simulink model "gm_uz_pmsm_model_9ph_vnl"  (R2021b)
settings: Solver=FixedStepAuto  StartTime=0.0  StopTime=0.8  RelTol=1e-3
PreLoadFcn:
  | uz_pmsm_model_9ph_init_parameter
undefined symbols (not defined in the file or in its folder): a, b, c, friction_coefficient, inertia, k_i_d, k_i_q, k_p_d, k_p_q, Kpd, L_d, L_o1, L_o2, L_q, L_x1, L_x2, L_y1, L_y2, L_zero, polepair, psi_pm, R_1, static_friction_torque, Tnd, ts
libraries: hdlmdlgenlib x191, hdlsllib x90, dspsigops x19, simulink x17, slpidlib x2, spsAlphaBetaZerotodq0Lib x1, pid_lib x1, spsdq0toAlphaBetaZeroLib x1
(part 6 of 7)

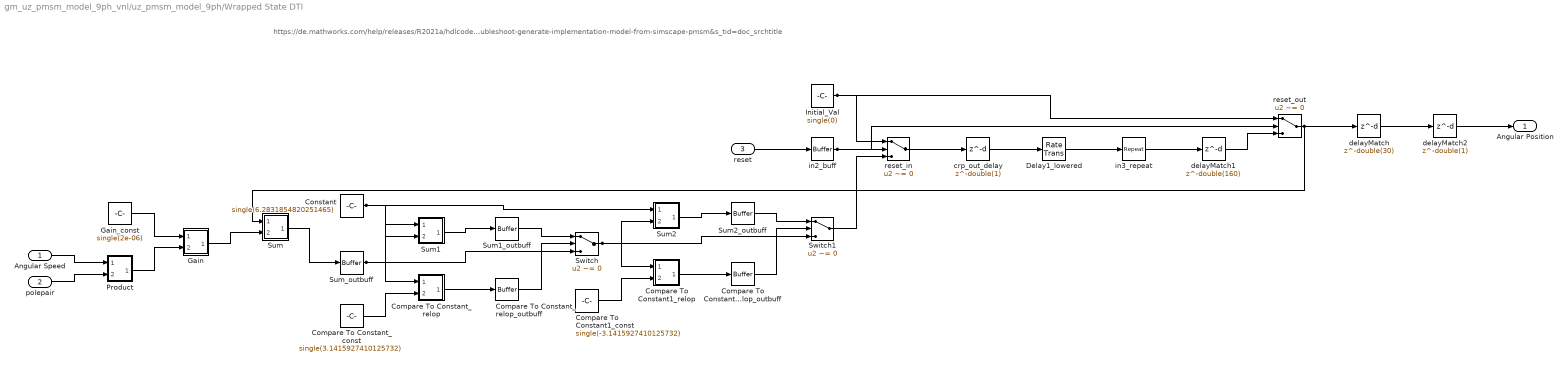
== system gm_uz_pmsm_model_9ph_vnl/uz_pmsm_model_9ph/Wrapped State DTI ==
  note: https://de.mathworks.com/help/releases/R2021a/hdlcoder/ug/troubleshoot-generate-implementation-model-from-simscape-pmsm.html?searchHighlight=troubleshoot-generate-implementation-model-from-simscape-pmsm&s_tid=doc_srchtitle
  Angular Speed : Inport  OutDataTypeStr=single  PortDimensions=1  SampleTime=1e-08
  polepair : Inport  Port=2  OutDataTypeStr=single  PortDimensions=1  SampleTime=1e-08
  reset : Inport  Port=3  OutDataTypeStr=boolean  PortDimensions=1  SampleTime=1e-08
  Compare To Constant1_const : Constant  Value=single(-3.1415927410125732)  OutDataTypeStr=single  SampleTime=1e-08
  Compare To Constant1_relop : Subsystem
      mask Display: disp('NFP\nrelop');
  Compare To Constant1_relop_outbuff : hdlmdlgenlib/Buffer
      settings: SourceProductBaseCode=SL
  Compare To Constant_const : Constant  Value=single(3.1415927410125732)  OutDataTypeStr=single  SampleTime=1e-08
  Compare To Constant_relop : Subsystem
      mask Display: disp('NFP\nrelop');
  Compare To Constant_relop_outbuff : hdlmdlgenlib/Buffer
      settings: SourceProductBaseCode=SL
  Constant : Constant  Value=single(6.2831854820251465)  OutDataTypeStr=single  SampleTime=1e-08
  Delay1_lowered : RateTransition  OutPortSampleTimeOpt=Multiple of input port sample time  OutPortSampleTimeMultiple=200
  Gain : Subsystem
      mask Display: disp('NFP\nmul');
  Gain_const : Constant  Value=single(2e-06)  OutDataTypeStr=single  SampleTime=1e-08
  Initial_Val : Constant  Value=single(0)  OutDataTypeStr=single  SampleTime=1e-08
  Product : Subsystem
      mask Display: disp('NFP\nmul');
  Sum : Subsystem
      mask Display: disp('NFP\nadd');
  Sum1 : Subsystem
      mask Display: disp('NFP\nadd');
  Sum1_outbuff : hdlmdlgenlib/Buffer
      settings: SourceProductBaseCode=SL
  Sum2 : Subsystem
      mask Display: disp('NFP\nadd');
  Sum2_outbuff : hdlmdlgenlib/Buffer
      settings: SourceProductBaseCode=SL
  Sum_outbuff : hdlmdlgenlib/Buffer
      settings: SourceProductBaseCode=SL
  Switch : Switch  Criteria=u2 ~= 0  Threshold=double(0)  OutDataTypeStr=single  SampleTime=1e-08
  Switch1 : Switch  Criteria=u2 ~= 0  Threshold=double(0)  OutDataTypeStr=single  SampleTime=1e-08
  crp_out_delay : Delay  DelayLength=double(1)  InitialCondition=0  SampleTime=1e-08
  delayMatch : Delay  DelayLength=double(30)  InitialCondition=0  SampleTime=1e-08
  delayMatch1 : Delay  DelayLength=double(160)  InitialCondition=0  SampleTime=1e-08
  delayMatch2 : Delay  DelayLength=double(1)  InitialCondition=0  SampleTime=1e-08
  in2_buff : hdlmdlgenlib/Buffer
      settings: SourceProductBaseCode=SL
  in3_repeat : dspsigops/Repeat  N=double(200)  RateOptions=Allow multirate processing  ic=0  mode=Unused parameter value
  reset_in : Switch  Criteria=u2 ~= 0  Threshold=double(0)  OutDataTypeStr=single  SampleTime=1e-08
  reset_out : Switch  Criteria=u2 ~= 0  Threshold=double(0)  OutDataTypeStr=single  SampleTime=1e-08
  Angular Position : Outport  SampleTime=1e-08
  wires:
  delayMatch/1 -> delayMatch2/1
  reset_out/1 -> Sum/1(In1), delayMatch/1
  Switch/1 -> Switch1/3, Compare To Constant1_relop/1(In1), Sum2/2(In2)
  Compare To Constant1_relop_outbuff/1 -> Switch1/2
  Sum_outbuff/1 -> Switch/3, Sum1/1(In1), Compare To Constant_relop/1(In1)
  Compare To Constant_relop_outbuff/1 -> Switch/2
  delayMatch1/1 -> reset_out/3
  in2_buff/1 -> reset_in/2, reset_out/2
  Gain/1(Out1) -> Sum/2(In2)
  Compare To Constant_relop/1(Out1) -> Compare To Constant_relop_outbuff/1
  Sum2/1(Out1) -> Sum2_outbuff/1
  Compare To Constant1_relop/1(Out1) -> Compare To Constant1_relop_outbuff/1
  Sum/1(Out1) -> Sum_outbuff/1
  Product/1(Out1) -> Gain/2(In2)
  Sum1/1(Out1) -> Sum1_outbuff/1
  Gain_const/1 -> Gain/1(In1)
  Compare To Constant_const/1 -> Compare To Constant_relop/2(In2)
  Compare To Constant1_const/1 -> Compare To Constant1_relop/2(In2)
  reset_in/1 -> crp_out_delay/1
  Sum2_outbuff/1 -> Switch1/1
  Switch1/1 -> reset_in/3
  Initial_Val/1 -> reset_in/1, reset_out/1
  Sum1_outbuff/1 -> Switch/1
  Constant/1 -> Sum1/2(In2), Sum2/1(In1)
  delayMatch2/1 -> Angular Position/1
  in3_repeat/1 -> delayMatch1/1
  crp_out_delay/1 -> Delay1_lowered/1
  Delay1_lowered/1 -> in3_repeat/1
  reset/1 -> in2_buff/1
  polepair/1 -> Product/2(In2)
  Angular Speed/1 -> Product/1(In1)

== system gm_uz_pmsm_model_9ph_vnl/uz_pmsm_model_9ph_vnl/Line-Line to Phase voltage ==
  In1 : Inport
  Complex to Real-Imag : ComplexToRealImag
  Constant : Constant  Value=0  OutDataTypeStr=single  SampleTime=ts
  Constant1 : Constant  Value=1/sqrt(3)*exp(1i*-30/180*pi)  OutDataTypeStr=single  SampleTime=ts
  Demux3 : Demux  Outputs=3
  Mux4 : Mux  Inputs=3
  Product : Product  OutDataTypeStr=single
  Real-Imag to Complex : RealImagToComplex
  Terminator : Terminator
  abc   to   alpha_beta_0 : Subsystem
  alpha_beta_0   to   abc : Subsystem
  Out1 : Outport
  wires:
  Constant1/1 -> Product/2
  alpha_beta_0   to   abc/1("a, b, c") -> Out1/1
  abc   to   alpha_beta_0/1("alpha, beta, 0 ") -> Demux3/1
  Demux3/3 -> Terminator/1
  In1/1 -> abc   to   alpha_beta_0/1("a, b, c")
  Constant/1 -> Mux4/3
  Complex to Real-Imag/2 -> Mux4/2
  Demux3/1 -> Real-Imag to Complex/1
  Real-Imag to Complex/1 -> Product/1
  Product/1 -> Complex to Real-Imag/1
  Mux4/1 -> alpha_beta_0   to   abc/1("alpha, beta, 0  ")
  Complex to Real-Imag/1 -> Mux4/1
  Demux3/2 -> Real-Imag to Complex/2

== system gm_uz_pmsm_model_9ph_vnl/uz_pmsm_model_9ph_vnl/Line-Line to Phase voltage1 ==
  In1 : Inport
  Complex to Real-Imag : ComplexToRealImag
  Constant : Constant  Value=0  OutDataTypeStr=single  SampleTime=ts
  Constant1 : Constant  Value=1/sqrt(3)*exp(1i*-30/180*pi)  OutDataTypeStr=single  SampleTime=ts
  Demux3 : Demux  Outputs=3
  Mux4 : Mux  Inputs=3
  Product : Product  OutDataTypeStr=single
  Real-Imag to Complex : RealImagToComplex
  Terminator : Terminator
  abc   to   alpha_beta_0 : Subsystem
  alpha_beta_0   to   abc : Subsystem
  Out1 : Outport
  wires:
  Demux3/2 -> Real-Imag to Complex/2
  Complex to Real-Imag/1 -> Mux4/1
  Mux4/1 -> alpha_beta_0   to   abc/1("alpha, beta, 0  ")
  Product/1 -> Complex to Real-Imag/1
  Real-Imag to Complex/1 -> Product/1
  Demux3/1 -> Real-Imag to Complex/1
  Complex to Real-Imag/2 -> Mux4/2
  Constant/1 -> Mux4/3
  In1/1 -> abc   to   alpha_beta_0/1("a, b, c")
  Demux3/3 -> Terminator/1
  abc   to   alpha_beta_0/1("alpha, beta, 0 ") -> Demux3/1
  alpha_beta_0   to   abc/1("a, b, c") -> Out1/1
  Constant1/1 -> Product/2

== system gm_uz_pmsm_model_9ph_vnl/uz_pmsm_model_9ph_vnl/Line-Line to Phase voltage2 ==
  In1 : Inport
  Complex to Real-Imag : ComplexToRealImag
  Constant : Constant  Value=0  OutDataTypeStr=single  SampleTime=ts
  Constant1 : Constant  Value=1/sqrt(3)*exp(1i*-30/180*pi)  OutDataTypeStr=single  SampleTime=ts
  Demux3 : Demux  Outputs=3
  Mux4 : Mux  Inputs=3
  Product : Product  OutDataTypeStr=single
  Real-Imag to Complex : RealImagToComplex
  Terminator : Terminator
  abc   to   alpha_beta_0 : Subsystem
  alpha_beta_0   to   abc : Subsystem
  Out1 : Outport
  wires:
  Constant1/1 -> Product/2
  alpha_beta_0   to   abc/1("a, b, c") -> Out1/1
  abc   to   alpha_beta_0/1("alpha, beta, 0 ") -> Demux3/1
  Demux3/3 -> Terminator/1
  In1/1 -> abc   to   alpha_beta_0/1("a, b, c")
  Constant/1 -> Mux4/3
  Complex to Real-Imag/2 -> Mux4/2
  Demux3/1 -> Real-Imag to Complex/1
  Real-Imag to Complex/1 -> Product/1
  Product/1 -> Complex to Real-Imag/1
  Mux4/1 -> alpha_beta_0   to   abc/1("alpha, beta, 0  ")
  Complex to Real-Imag/1 -> Mux4/1
  Demux3/2 -> Real-Imag to Complex/2

== system gm_uz_pmsm_model_9ph_vnl/uz_pmsm_model_9ph_vnl/Transformation ==
  in : Inport
  Add : Sum
  Add1 : Sum  Inputs=-+
  Constant1 : Constant  Value=c  OutDataTypeStr=fixdt(1,18)  SampleTime=ts
  Data Type Conversion1 : DataTypeConversion  OutDataTypeStr=single  RndMeth=Nearest
  Data Type Conversion38 : DataTypeConversion  OutDataTypeStr=single  RndMeth=Nearest
  Data Type Conversion39 : DataTypeConversion  OutDataTypeStr=single  RndMeth=Nearest
  Demux1 : Demux  Outputs=9
  Divide{,1..3} (4 alike) : Product  Inputs=**
  MatrixMultiply : Product  Multiplication=Matrix(*)
  Mux : Mux  Inputs=9
  out : Outport
  wires:
  in/1 -> MatrixMultiply/2
  Data Type Conversion39/1 -> Demux1/1
  Constant1/1 -> MatrixMultiply/1
  MatrixMultiply/1 -> Data Type Conversion39/1
  Divide2/1 -> Add1/1
  Divide3/1 -> Add1/2
  [cos_theta_el] -> Divide3/1
  [sin_theta_el] -> Divide2/1
  [cos_theta_el] -> Divide/1  "cos_theta_hdl"
  [sin_theta_el] -> Divide1/1  "sin_theta_hdl"
  Divide1/1 -> Add/2
  Divide/1 -> Add/1
  Data Type Conversion1/1 -> Divide3/2, Divide1/2  "u_beta"
  Data Type Conversion38/1 -> Divide2/2, Divide/2  "u_alpha"
  Add/1 -> Mux/1
  Add1/1 -> Mux/2
  Demux1/2 -> Data Type Conversion1/1
  Demux1/1 -> Data Type Conversion38/1
  Mux/1 -> out/1  "trafo_out"
  Demux1/9 -> Mux/9
  Demux1/8 -> Mux/8
  Demux1/7 -> Mux/7
  Demux1/6 -> Mux/6
  Demux1/5 -> Mux/5
  Demux1/4 -> Mux/4
  Demux1/3 -> Mux/3

== system gm_uz_pmsm_model_9ph_vnl/uz_pmsm_model_9ph_vnl/Transformation1 ==
  in : Inport
  Add : Sum  Inputs=+-
  Add1 : Sum
  Constant1 : Constant  Value=inv(c)  OutDataTypeStr=fixdt(1,18)  SampleTime=ts
  Data Type Conversion28 : DataTypeConversion  OutDataTypeStr=fixdt(1,25,12)  RndMeth=Nearest
  Demux1 : Demux  Outputs=9
  Divide{,1..3} (4 alike) : Product  Inputs=**
  MatrixMultiply : Product  Multiplication=Matrix(*)
  Mux : Mux  Inputs=9
  out : Outport
  wires:
  MatrixMultiply/1 -> out/1
  Constant1/1 -> MatrixMultiply/1
  Data Type Conversion28/1 -> MatrixMultiply/2
  Add1/1 -> Mux/2
  [cos_theta_el] -> Divide3/1
  Divide2/1 -> Add1/1
  [sin_theta_el] -> Divide2/1
  Divide3/1 -> Add1/2
  Demux1/1 -> Divide/2, Divide2/2  "i_d"
  Divide1/1 -> Add/2
  [cos_theta_el] -> Divide/1
  Divide/1 -> Add/1
  Add/1 -> Mux/1
  Demux1/2 -> Divide1/2, Divide3/2  "i_q"
  [sin_theta_el] -> Divide1/1
  Demux1/7 -> Mux/7
  Demux1/9 -> Mux/9
  Demux1/5 -> Mux/5
  Demux1/3 -> Mux/3
  Demux1/4 -> Mux/4
  Demux1/6 -> Mux/6
  Demux1/8 -> Mux/8
  Mux/1 -> Data Type Conversion28/1
  in/1 -> Demux1/1

== system gm_uz_pmsm_model_9ph_vnl/uz_pmsm_model_9ph_vnl/Wrapped State DTI ==
  note: https://de.mathworks.com/help/releases/R2021a/hdlcoder/ug/troubleshoot-generate-implementation-model-from-simscape-pmsm.html?searchHighlight=troubleshoot-generate-implementation-model-from-simscape-pmsm&s_tid=doc_srchtitle
  Angular Speed : Inport
  polepair : Inport  Port=2
  reset : Inport  Port=3
  Compare To Constant : simulink/Logic and Bit Operations/Compare To Constant  relop=>=  const=single(pi)  OutDataTypeStr=boolean
  Compare To Constant1 : simulink/Logic and Bit Operations/Compare To Constant  relop=<  const=single(-pi)  OutDataTypeStr=boolean
  Constant : Constant  Value=single(2*pi)  SampleTime=-1
  Delay1 : Delay  DelayLength=1  ExternalReset=Level
      settings: InputPortMap=u0,r5
  Gain : Gain  Gain=ts
  Product : Product
  Sum : Sum  Inputs=|++
  Sum1 : Sum  Inputs=|-+
  Sum2 : Sum  Inputs=|++
  Switch : Switch  Criteria=u2 > Threshold
  Switch1 : Switch  Criteria=u2 > Threshold
  Angular Position : Outport
  wires:
  polepair/1 -> Product/2
  Angular Speed/1 -> Product/1
  Product/1 -> Gain/1
  reset/1 -> Delay1/2
  Gain/1 -> Sum/2
  Sum1/1 -> Switch/1
  Sum/1 -> Switch/3, Sum1/2, Compare To Constant/1
  Compare To Constant/1 -> Switch/2
  Switch/1 -> Switch1/3, Compare To Constant1/1, Sum2/2
  Switch1/1 -> Delay1/1  "Angular Position"
  Sum2/1 -> Switch1/1
  Constant/1 -> Sum1/1, Sum2/1
  Delay1/1 -> Angular Position/1, Sum/1
  Compare To Constant1/1 -> Switch1/2

== system gm_uz_pmsm_model_9ph_vnl/uz_pmsm_model_9ph_vnl/mechanical_system ==
  note: This delay breaks the algebraic loop between mechanical and electrical system.
      | Introduces a delay of 500ns.
  note: load torque negative!!!
  reset : Inport
  M_Mi : Inport  Port=2
  reciprocal_J : Inport  Port=3
  load_torque : Inport  Port=4
  Data Type Conversion1 : DataTypeConversion  OutDataTypeStr=double  RndMeth=Nearest
  Data Type Conversion8 : DataTypeConversion  OutDataTypeStr=single  RndMeth=Nearest
  Delay : Delay  DelayLength=1
  Product11 : Product
  Sum1 : Sum  Inputs=|++
  integrator : Subsystem
  omega_mech : Outport
  wires:
  reset/1 -> integrator/2(reset)
  Data Type Conversion1/1 -> integrator/1(in)
  Data Type Conversion8/1 -> omega_mech/1
  Delay/1 -> Sum1/1
  M_Mi/1 -> Delay/1
  load_torque/1 -> Sum1/2
  Sum1/1 -> Product11/2
  reciprocal_J/1 -> Product11/1
  integrator/1(outt) -> Data Type Conversion8/1
  Product11/1 -> Data Type Conversion1/1

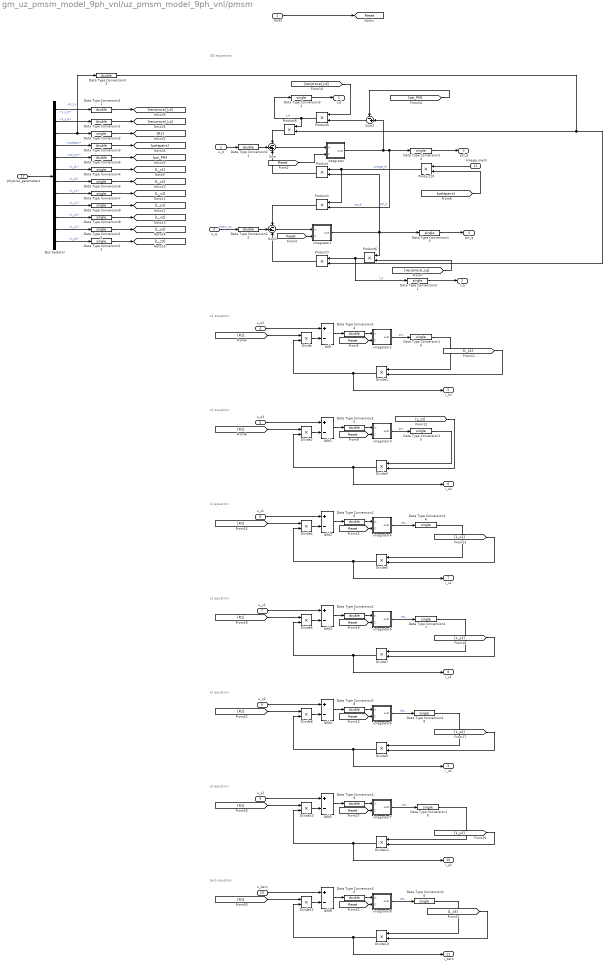
== system gm_uz_pmsm_model_9ph_vnl/uz_pmsm_model_9ph_vnl/pmsm ==
  note: zero equation
  note: y2 equation
  note: x2 equation
  note: y1 equation
  note: x1 equation
  note: o2 equation
  note: DQ equations
  note: o1 equation
  reset : Inport
  u_d : Inport  Port=2
  u_q : Inport  Port=3
  u_o1 : Inport  Port=4
  u_o2 : Inport  Port=5
  u_x1 : Inport  Port=6
  u_y1 : Inport  Port=7
  u_x2 : Inport  Port=8
  u_y2 : Inport  Port=9
  u_zero : Inport  Port=10
  omega_mech : Inport  Port=11
  physical_parameters : Inport  Port=12
  Add{,1..6} (7 alike) : Sum  Inputs=+-
  Bus Selector : BusSelector  OutputSignals=1_L_d,1_L_q,R_1,polepair,psi_pm,L_z1,L_z2,L_x1,L_y1,L_x2,L_y2,L_z3
  Data Type Conversion{1,3,5,11,21..22,24..30,33} (14 alike) : DataTypeConversion  OutDataTypeStr=double  RndMeth=Nearest
  Data Type Conversion{2,4,6..10,12..20,23,31..32} (19 alike) : DataTypeConversion  OutDataTypeStr=single  RndMeth=Nearest
  Divide{,1..13} (14 alike) : Product  Inputs=**
  Product{,1,5..8,10} (7 alike) : Product
  Sum : Sum  Inputs=-++
  Sum1 : Sum  Inputs=-+-
  Sum2 : Sum  Inputs=-+|
  integrator : Subsystem
  integrator1 : Subsystem
  integrator2 : Subsystem
  integrator3 : Subsystem
  integrator4 : Subsystem
  integrator5 : Subsystem
  integrator6 : Subsystem
  integrator7 : Subsystem
  integrator8 : Subsystem
  I_d : Outport
  I_q : Outport  Port=2
  psi_d : Outport  Port=3
  psi_q : Outport  Port=4
  i_o1 : Outport  Port=5
  i_o2 : Outport  Port=6
  i_x1 : Outport  Port=7
  i_y1 : Outport  Port=8
  i_x2 : Outport  Port=9
  i_y2 : Outport  Port=10
  i_zero : Outport  Port=11
  tag scope: Reset=global
  wires:
  Data Type Conversion32/1 -> I_d/1
  Data Type Conversion23/1 -> psi_d/1
  Data Type Conversion21/1 -> Sum/2
  Data Type Conversion31/1 -> I_q/1
  Data Type Conversion13/1 -> psi_q/1
  Data Type Conversion22/1 -> Sum1/2
  Data Type Conversion30/1 -> integrator8/1(in)
  Data Type Conversion29/1 -> integrator7/1(in)
  Data Type Conversion28/1 -> integrator6/1(in)
  Data Type Conversion27/1 -> integrator5/1(in)
  Data Type Conversion26/1 -> integrator4/1(in)
  Data Type Conversion25/1 -> integrator3/1(in)
  Data Type Conversion24/1 -> integrator2/1(in)
  Sum1/1 -> integrator1/1(in)
  Sum/1 -> integrator/1(in)
  Data Type Conversion20/1 -> Divide13/1
  Data Type Conversion19/1 -> Divide11/1
  Data Type Conversion18/1 -> Divide9/1
  Data Type Conversion17/1 -> Divide7/1
  Data Type Conversion16/1 -> Divide5/1
  Data Type Conversion15/1 -> Divide3/1
  Data Type Conversion14/1 -> Divide1/1
  [L_z3] -> Divide13/2
  [L_y2] -> Divide11/2
  [L_x2] -> Divide9/2
  [L_y1] -> Divide7/2
  [L_x1] -> Divide5/2
  [polepairs] -> Product10/2
  Data Type Conversion2/1 -> [R1]
  Bus Selector/9 -> Data Type Conversion9/1  "<L_y1>"
  Data Type Conversion11/1 -> [reciprocal_Ld]
  Data Type Conversion3/1 -> [polepairs]
  physical_parameters/1 -> Bus Selector/1
  Data Type Conversion4/1 -> [L_z1]
  Bus Selector/10 -> Data Type Conversion8/1  "<L_x2>"
  Bus Selector/3 -> Data Type Conversion2/1, Data Type Conversion33/1  "<R_1>"
  Bus Selector/12 -> Data Type Conversion12/1  "<L_z3>"
  Bus Selector/11 -> Data Type Conversion10/1  "<L_y2>"
  Data Type Conversion6/1 -> [L_z2]
  Data Type Conversion7/1 -> [L_x1]
  Bus Selector/7 -> Data Type Conversion6/1  "<L_z2>"
  Bus Selector/6 -> Data Type Conversion4/1  "<L_z1>"
  Data Type Conversion10/1 -> [L_y2]
  Data Type Conversion8/1 -> [L_x2]
  Bus Selector/5 -> Data Type Conversion5/1  "<psi_pm>"
  Bus Selector/2 -> Data Type Conversion1/1  "<1_L_q>"
  Bus Selector/8 -> Data Type Conversion7/1  "<L_x1>"
  Bus Selector/4 -> Data Type Conversion3/1  "<polepair>"
  Data Type Conversion5/1 -> [psi_PM]
  Data Type Conversion1/1 -> [reciprocal_Lq]
  Data Type Conversion9/1 -> [L_y1]
  Data Type Conversion12/1 -> [L_z3]
  Bus Selector/1 -> Data Type Conversion11/1  "<1_L_d>"
  integrator8/1(outt) -> Data Type Conversion20/1  "psi_"
  [R1] -> Divide12/1
  Add6/1 -> Data Type Conversion30/1
  Divide12/1 -> Add6/2
  Divide13/1 -> Divide12/2, i_zero/1
  u_zero/1 -> Add6/1
  [Reset] -> integrator8/2(reset)
  [Reset] -> integrator7/2(reset)
  u_y2/1 -> Add5/1
  Divide11/1 -> Divide10/2, i_y2/1
  Divide10/1 -> Add5/2
  Add5/1 -> Data Type Conversion29/1
  [R1] -> Divide10/1
  integrator7/1(outt) -> Data Type Conversion19/1  "psi_"
  integrator6/1(outt) -> Data Type Conversion18/1  "psi_"
  [R1] -> Divide8/1
  Add4/1 -> Data Type Conversion28/1
  Divide8/1 -> Add4/2
  Divide9/1 -> Divide8/2, i_x2/1
  u_x2/1 -> Add4/1
  [Reset] -> integrator6/2(reset)
  [Reset] -> integrator5/2(reset)
  u_y1/1 -> Add3/1
  Divide7/1 -> Divide6/2, i_y1/1
  Divide6/1 -> Add3/2
  Add3/1 -> Data Type Conversion27/1
  [R1] -> Divide6/1
  integrator5/1(outt) -> Data Type Conversion17/1  "psi_"
  integrator4/1(outt) -> Data Type Conversion16/1  "psi_"
  [R1] -> Divide4/1
  Add2/1 -> Data Type Conversion26/1
  Divide4/1 -> Add2/2
  Divide5/1 -> Divide4/2, i_x1/1
  u_x1/1 -> Add2/1
  [Reset] -> integrator4/2(reset)
  [Reset] -> integrator3/2(reset)
  [L_z2] -> Divide3/2
  u_o2/1 -> Add1/1
  Divide3/1 -> Divide2/2, i_o2/1
  Divide2/1 -> Add1/2
  Add1/1 -> Data Type Conversion25/1
  [R1] -> Divide2/1
  integrator3/1(outt) -> Data Type Conversion15/1  "psi_"
  integrator2/1(outt) -> Data Type Conversion14/1  "psi_"
  [R1] -> Divide/1
  Add/1 -> Data Type Conversion24/1
  Divide/1 -> Add/2
  Divide1/1 -> Divide/2, i_o1/1
  u_o1/1 -> Add/1
  [L_z1] -> Divide1/2
  [Reset] -> integrator2/2(reset)
  [Reset] -> integrator1/2(reset)
  [Reset] -> integrator/2(reset)
  reset/1 -> [Reset]
  Data Type Conversion33/1 -> Product7/2, Product8/2
  Product7/1 -> Sum1/3
  [reciprocal_Lq] -> Product6/2
  Product8/1 -> Sum/1
  Sum2/1 -> Product5/2
  integrator/1(outt) -> Data Type Conversion23/1, Product1/2, Sum2/2  "psi_d"
  Product10/1 -> Product/1, Product1/1  "omega_el"
  Product6/1 -> Product7/1, Data Type Conversion31/1  "I_q"
  [psi_PM] -> Sum2/1
  Product1/1 -> Sum1/1
  u_d/1 -> Data Type Conversion21/1
  integrator1/1(outt) -> Product6/1, Product/2, Data Type Conversion13/1  "psi_q"
  [reciprocal_Ld] -> Product5/1
  Product5/1 -> Product8/1, Data Type Conversion32/1  "I_d"
  Product/1 -> Sum/3
  u_q/1 -> Data Type Conversion22/1  "intern_uq"
  omega_mech/1 -> Product10/1

== system gm_uz_pmsm_model_9ph_vnl/uz_pmsm_model_9ph_vnl/torque_calculation ==
  I_d : Inport
  I_q : Inport  Port=2
  psi_d : Inport  Port=3
  psi_q : Inport  Port=4
  polepairs : Inport  Port=5
  Factor : Gain  Gain=9/2
  Product2 : Product
  Product3 : Product
  Product9 : Product
  Sum3 : Sum  Inputs=-|+
  M_Mi : Outport
  wires:
  Factor/1 -> Product9/1  "M_Mi"
  polepairs/1 -> Product9/2
  Product9/1 -> M_Mi/1  "M_Mi"
  I_q/1 -> Product3/2
  I_d/1 -> Product2/1
  psi_d/1 -> Product3/1
  psi_q/1 -> Product2/2
  Product2/1 -> Sum3/1
  Product3/1 -> Sum3/2
  Sum3/1 -> Factor/1

== system gm_uz_pmsm_model_9ph_vnl/Compare/Assert_i_abc_ps/RelErrCheck ==
  In1 : Inport
  In2 : Inport  Port=2
  "RelativeErrorCheck " : MATLAB Function  TreatAsAtomicUnit=on
  Out1 : Outport  VectorParamsAs1DForOutWhenUnconnected=off
  wires:
  "RelativeErrorCheck "/1(y) -> Out1/1
  In1/1 -> "RelativeErrorCheck "/1(P)
  In2/1 -> "RelativeErrorCheck "/2(R)

== system gm_uz_pmsm_model_9ph_vnl/Compare/Assert_outputs/RelErrCheck ==
  In1 : Inport
  In2 : Inport  Port=2
  "RelativeErrorCheck " : MATLAB Function  TreatAsAtomicUnit=on
  Out1 : Outport  VectorParamsAs1DForOutWhenUnconnected=off
  wires:
  "RelativeErrorCheck "/1(y) -> Out1/1
  In1/1 -> "RelativeErrorCheck "/1(P)
  In2/1 -> "RelativeErrorCheck "/2(R)

== system gm_uz_pmsm_model_9ph_vnl/uz_pmsm_model_9ph/Line-Line to Phase voltage/Product ==
  In1 : Inport
  In2 : Inport  Port=2
  Product : Product  Inputs=**  OutDataTypeStr=single  SampleTime=1e-08
  Product_pd1 : Delay  DelayLength=6
  Out1 : Outport
  wires:
  Product_pd1/1 -> Out1/1
  Product/1 -> Product_pd1/1
  In2/1 -> Product/2
  In1/1 -> Product/1

== system gm_uz_pmsm_model_9ph_vnl/uz_pmsm_model_9ph/Line-Line to Phase voltage/Product1 ==
  In1 : Inport
  In2 : Inport  Port=2
  Product1 : Product  Inputs=**  OutDataTypeStr=single  SampleTime=1e-08
  Product1_pd1 : Delay  DelayLength=6
  Out1 : Outport
  wires:
  Product1_pd1/1 -> Out1/1
  Product1/1 -> Product1_pd1/1
  In2/1 -> Product1/2
  In1/1 -> Product1/1

== system gm_uz_pmsm_model_9ph_vnl/uz_pmsm_model_9ph/Line-Line to Phase voltage/Product2 ==
  In1 : Inport
  In2 : Inport  Port=2
  Product2 : Product  Inputs=**  OutDataTypeStr=single  SampleTime=1e-08
  Product2_pd1 : Delay  DelayLength=6
  Out1 : Outport
  wires:
  Product2_pd1/1 -> Out1/1
  Product2/1 -> Product2_pd1/1
  In2/1 -> Product2/2
  In1/1 -> Product2/1

== system gm_uz_pmsm_model_9ph_vnl/uz_pmsm_model_9ph/Line-Line to Phase voltage/Product3 ==
  In1 : Inport
  In2 : Inport  Port=2
  Product3 : Product  Inputs=**  OutDataTypeStr=single  SampleTime=1e-08
  Product3_pd1 : Delay  DelayLength=6
  Out1 : Outport
  wires:
  Product3_pd1/1 -> Out1/1
  Product3/1 -> Product3_pd1/1
  In2/1 -> Product3/2
  In1/1 -> Product3/1

== system gm_uz_pmsm_model_9ph_vnl/uz_pmsm_model_9ph/Line-Line to Phase voltage/Product_AC_minus_BD ==
  In1 : Inport
  In2 : Inport  Port=2
  Product_AC_minus_BD : Sum  Inputs=+-  OutDataTypeStr=single  SampleTime=1e-08
  Product_AC_minus_BD_pd1 : Delay  DelayLength=6
  Out1 : Outport
  wires:
  Product_AC_minus_BD_pd1/1 -> Out1/1
  Product_AC_minus_BD/1 -> Product_AC_minus_BD_pd1/1
  In2/1 -> Product_AC_minus_BD/2
  In1/1 -> Product_AC_minus_BD/1

== system gm_uz_pmsm_model_9ph_vnl/uz_pmsm_model_9ph/Line-Line to Phase voltage/Product_AD_plus_BC ==
  In1 : Inport
  In2 : Inport  Port=2
  Product_AD_plus_BC : Sum  OutDataTypeStr=single  SampleTime=1e-08
  Product_AD_plus_BC_pd1 : Delay  DelayLength=6
  Out1 : Outport
  wires:
  Product_AD_plus_BC_pd1/1 -> Out1/1
  Product_AD_plus_BC/1 -> Product_AD_plus_BC_pd1/1
  In2/1 -> Product_AD_plus_BC/2
  In1/1 -> Product_AD_plus_BC/1

== system gm_uz_pmsm_model_9ph_vnl/uz_pmsm_model_9ph/Line-Line to Phase voltage/abc   to   alpha_beta_0 ==
  "a, b, c" : Inport  OutDataTypeStr=single  PortDimensions=[3]  SampleTime=1e-08
  Gain2 : Subsystem
      mask Display: disp('NFP\nmul');
  Gain2_const : Constant  Value=single(0.6666666865348816)  OutDataTypeStr=single  SampleTime=1e-08
  Gain4_const : Constant  Value=single([1 0 0.5 -0.5 0.8660253882408142 0.5 -0.5 -0.8660253882408142 0.5]).'  OutDataTypeStr=single  SampleTime=1e-08
  MMul_add_01 : Subsystem
      mask Display: disp('NFP\nadd');
  MMul_add_12 : Subsystem
      mask Display: disp('NFP\nadd');
  MMul_dot_product : Subsystem
      mask Display: disp('NFP\nmul');
  Reshape : Reshape  OutputDimensionality=Column vector (2-D)
  Row2Col_in0 : Reshape  OutputDimensionality=Column vector (2-D)
  Row2Col_in1 : Reshape  OutputDimensionality=Column vector (2-D)
  delayMatch : Delay  DelayLength=double(6)  InitialCondition=0  SampleTime=1e-08
  delayMatch1 : Delay  DelayLength=double(18)  InitialCondition=0  SampleTime=1e-08
  reshape_dotProduct : Reshape  OutputDimensionality=Customize  OutputDimensions=[3,3]
  reshape_mmulResult : Reshape  OutputDimensionality=Customize  OutputDimensions=[3,1]
  select_0 : Selector  NumberOfDimensions=2  SampleTime=1e-08  IndexOptions=Index vector (dialog),Select all  Indices=double(1),[]  OutputSizes=1
  select_1 : Selector  NumberOfDimensions=2  SampleTime=1e-08  IndexOptions=Index vector (dialog),Select all  Indices=double(2),[]  OutputSizes=1
  select_2 : Selector  NumberOfDimensions=2  SampleTime=1e-08  IndexOptions=Index vector (dialog),Select all  Indices=double(3),[]  OutputSizes=1
  select_indices0 : Selector  SampleTime=1e-08  IndexOptions=Index vector (dialog)  Indices=double([1 4 7 2 5 8 3 6 9])  OutputSizes=1
  select_indices1 : Selector  SampleTime=1e-08  IndexOptions=Index vector (dialog)  Indices=double([1 2 3 1 2 3 1 2 3])  OutputSizes=1
  t : Reshape  OutputDimensionality=Customize  OutputDimensions=[3,3]
  t1 : Mux  Inputs=3
  vectorized_in0 : Reshape  OutputDimensionality=Row vector (2-D)
  "alpha, beta, 0 " : Outport  SampleTime=1e-08
  wires:
  "a, b, c"/1 -> Reshape/1
  t1/1 -> delayMatch1/1
  select_2/1 -> delayMatch/1
  Gain2/1(Out1) -> "alpha, beta, 0 "/1
  delayMatch1/1 -> Gain2/2(In2)
  MMul_add_12/1(Out1) -> reshape_mmulResult/1
  MMul_add_01/1(Out1) -> MMul_add_12/1(In1)
  MMul_dot_product/1(Out1) -> reshape_dotProduct/1
  Gain2_const/1 -> t1/1, t1/2, t1/3
  Gain4_const/1 -> t/1
  delayMatch/1 -> MMul_add_12/2(In2)
  select_1/1 -> MMul_add_01/2(In2)
  select_0/1 -> MMul_add_01/1(In1)
  reshape_dotProduct/1 -> select_0/1, select_1/1, select_2/1
  Row2Col_in1/1 -> MMul_dot_product/2(In2)
  Row2Col_in0/1 -> MMul_dot_product/1(In1)
  select_indices1/1 -> Row2Col_in1/1
  select_indices0/1 -> Row2Col_in0/1
  vectorized_in0/1 -> select_indices0/1
  t/1 -> vectorized_in0/1
  Reshape/1 -> select_indices1/1
  reshape_mmulResult/1 -> Gain2/1(In1)

== system gm_uz_pmsm_model_9ph_vnl/uz_pmsm_model_9ph/Line-Line to Phase voltage/alpha_beta_0   to   abc ==
  "alpha, beta, 0  " : Inport  OutDataTypeStr=single  PortDimensions=[3]  SampleTime=1e-08
  Gain4_const : Constant  Value=single([1 -0.5 -0.5 0 0.8660253882408142 -0.8660253882408142 1 1 1]).'  OutDataTypeStr=single  SampleTime=1e-08
  MMul_add_01 : Subsystem
      mask Display: disp('NFP\nadd');
  MMul_add_12 : Subsystem
      mask Display: disp('NFP\nadd');
  MMul_dot_product : Subsystem
      mask Display: disp('NFP\nmul');
  Reshape : Reshape  OutputDimensionality=Column vector (2-D)
  Row2Col_in0 : Reshape  OutputDimensionality=Column vector (2-D)
  Row2Col_in1 : Reshape  OutputDimensionality=Column vector (2-D)
  delayMatch : Delay  DelayLength=double(6)  InitialCondition=0  SampleTime=1e-08
  reshape_dotProduct : Reshape  OutputDimensionality=Customize  OutputDimensions=[3,3]
  reshape_mmulResult : Reshape  OutputDimensionality=Customize  OutputDimensions=[3,1]
  select_0 : Selector  NumberOfDimensions=2  SampleTime=1e-08  IndexOptions=Index vector (dialog),Select all  Indices=double(1),[]  OutputSizes=1
  select_1 : Selector  NumberOfDimensions=2  SampleTime=1e-08  IndexOptions=Index vector (dialog),Select all  Indices=double(2),[]  OutputSizes=1
  select_2 : Selector  NumberOfDimensions=2  SampleTime=1e-08  IndexOptions=Index vector (dialog),Select all  Indices=double(3),[]  OutputSizes=1
  select_indices0 : Selector  SampleTime=1e-08  IndexOptions=Index vector (dialog)  Indices=double([1 4 7 2 5 8 3 6 9])  OutputSizes=1
  select_indices1 : Selector  SampleTime=1e-08  IndexOptions=Index vector (dialog)  Indices=double([1 2 3 1 2 3 1 2 3])  OutputSizes=1
  t : Reshape  OutputDimensionality=Customize  OutputDimensions=[3,3]
  vectorized_in0 : Reshape  OutputDimensionality=Row vector (2-D)
  "a, b, c" : Outport  SampleTime=1e-08
  wires:
  "alpha, beta, 0  "/1 -> Reshape/1
  select_2/1 -> delayMatch/1
  MMul_add_12/1(Out1) -> reshape_mmulResult/1
  MMul_add_01/1(Out1) -> MMul_add_12/1(In1)
  MMul_dot_product/1(Out1) -> reshape_dotProduct/1
  Gain4_const/1 -> t/1
  delayMatch/1 -> MMul_add_12/2(In2)
  select_1/1 -> MMul_add_01/2(In2)
  select_0/1 -> MMul_add_01/1(In1)
  reshape_dotProduct/1 -> select_0/1, select_1/1, select_2/1
  Row2Col_in1/1 -> MMul_dot_product/2(In2)
  Row2Col_in0/1 -> MMul_dot_product/1(In1)
  select_indices1/1 -> Row2Col_in1/1
  select_indices0/1 -> Row2Col_in0/1
  vectorized_in0/1 -> select_indices0/1
  t/1 -> vectorized_in0/1
  Reshape/1 -> select_indices1/1
  reshape_mmulResult/1 -> "a, b, c"/1

== system gm_uz_pmsm_model_9ph_vnl/uz_pmsm_model_9ph/Line-Line to Phase voltage1/Product ==
  In1 : Inport
  In2 : Inport  Port=2
  Product : Product  Inputs=**  OutDataTypeStr=single  SampleTime=1e-08
  Product_pd1 : Delay  DelayLength=6
  Out1 : Outport
  wires:
  Product_pd1/1 -> Out1/1
  Product/1 -> Product_pd1/1
  In2/1 -> Product/2
  In1/1 -> Product/1

== system gm_uz_pmsm_model_9ph_vnl/uz_pmsm_model_9ph/Line-Line to Phase voltage1/Product1 ==
  In1 : Inport
  In2 : Inport  Port=2
  Product1 : Product  Inputs=**  OutDataTypeStr=single  SampleTime=1e-08
  Product1_pd1 : Delay  DelayLength=6
  Out1 : Outport
  wires:
  Product1_pd1/1 -> Out1/1
  Product1/1 -> Product1_pd1/1
  In2/1 -> Product1/2
  In1/1 -> Product1/1

== system gm_uz_pmsm_model_9ph_vnl/uz_pmsm_model_9ph/Line-Line to Phase voltage1/Product2 ==
  In1 : Inport
  In2 : Inport  Port=2
  Product2 : Product  Inputs=**  OutDataTypeStr=single  SampleTime=1e-08
  Product2_pd1 : Delay  DelayLength=6
  Out1 : Outport
  wires:
  Product2_pd1/1 -> Out1/1
  Product2/1 -> Product2_pd1/1
  In2/1 -> Product2/2
  In1/1 -> Product2/1

== system gm_uz_pmsm_model_9ph_vnl/uz_pmsm_model_9ph/Line-Line to Phase voltage1/Product3 ==
  In1 : Inport
  In2 : Inport  Port=2
  Product3 : Product  Inputs=**  OutDataTypeStr=single  SampleTime=1e-08
  Product3_pd1 : Delay  DelayLength=6
  Out1 : Outport
  wires:
  Product3_pd1/1 -> Out1/1
  Product3/1 -> Product3_pd1/1
  In2/1 -> Product3/2
  In1/1 -> Product3/1

== system gm_uz_pmsm_model_9ph_vnl/uz_pmsm_model_9ph/Line-Line to Phase voltage1/Product_AC_minus_BD ==
  In1 : Inport
  In2 : Inport  Port=2
  Product_AC_minus_BD : Sum  Inputs=+-  OutDataTypeStr=single  SampleTime=1e-08
  Product_AC_minus_BD_pd1 : Delay  DelayLength=6
  Out1 : Outport
  wires:
  Product_AC_minus_BD_pd1/1 -> Out1/1
  Product_AC_minus_BD/1 -> Product_AC_minus_BD_pd1/1
  In2/1 -> Product_AC_minus_BD/2
  In1/1 -> Product_AC_minus_BD/1

== system gm_uz_pmsm_model_9ph_vnl/uz_pmsm_model_9ph/Line-Line to Phase voltage1/Product_AD_plus_BC ==
  In1 : Inport
  In2 : Inport  Port=2
  Product_AD_plus_BC : Sum  OutDataTypeStr=single  SampleTime=1e-08
  Product_AD_plus_BC_pd1 : Delay  DelayLength=6
  Out1 : Outport
  wires:
  Product_AD_plus_BC_pd1/1 -> Out1/1
  Product_AD_plus_BC/1 -> Product_AD_plus_BC_pd1/1
  In2/1 -> Product_AD_plus_BC/2
  In1/1 -> Product_AD_plus_BC/1

== system gm_uz_pmsm_model_9ph_vnl/uz_pmsm_model_9ph/Line-Line to Phase voltage1/abc   to   alpha_beta_0 ==
  "a, b, c" : Inport  OutDataTypeStr=single  PortDimensions=[3]  SampleTime=1e-08
  Gain2 : Subsystem
      mask Display: disp('NFP\nmul');
  Gain2_const : Constant  Value=single(0.6666666865348816)  OutDataTypeStr=single  SampleTime=1e-08
  Gain4_const : Constant  Value=single([1 0 0.5 -0.5 0.8660253882408142 0.5 -0.5 -0.8660253882408142 0.5]).'  OutDataTypeStr=single  SampleTime=1e-08
  MMul_add_01 : Subsystem
      mask Display: disp('NFP\nadd');
  MMul_add_12 : Subsystem
      mask Display: disp('NFP\nadd');
  MMul_dot_product : Subsystem
      mask Display: disp('NFP\nmul');
  Reshape : Reshape  OutputDimensionality=Column vector (2-D)
  Row2Col_in0 : Reshape  OutputDimensionality=Column vector (2-D)
  Row2Col_in1 : Reshape  OutputDimensionality=Column vector (2-D)
  delayMatch : Delay  DelayLength=double(6)  InitialCondition=0  SampleTime=1e-08
  delayMatch1 : Delay  DelayLength=double(18)  InitialCondition=0  SampleTime=1e-08
  reshape_dotProduct : Reshape  OutputDimensionality=Customize  OutputDimensions=[3,3]
  reshape_mmulResult : Reshape  OutputDimensionality=Customize  OutputDimensions=[3,1]
  select_0 : Selector  NumberOfDimensions=2  SampleTime=1e-08  IndexOptions=Index vector (dialog),Select all  Indices=double(1),[]  OutputSizes=1
  select_1 : Selector  NumberOfDimensions=2  SampleTime=1e-08  IndexOptions=Index vector (dialog),Select all  Indices=double(2),[]  OutputSizes=1
  select_2 : Selector  NumberOfDimensions=2  SampleTime=1e-08  IndexOptions=Index vector (dialog),Select all  Indices=double(3),[]  OutputSizes=1
  select_indices0 : Selector  SampleTime=1e-08  IndexOptions=Index vector (dialog)  Indices=double([1 4 7 2 5 8 3 6 9])  OutputSizes=1
  select_indices1 : Selector  SampleTime=1e-08  IndexOptions=Index vector (dialog)  Indices=double([1 2 3 1 2 3 1 2 3])  OutputSizes=1
  t : Reshape  OutputDimensionality=Customize  OutputDimensions=[3,3]
  t1 : Mux  Inputs=3
  vectorized_in0 : Reshape  OutputDimensionality=Row vector (2-D)
  "alpha, beta, 0 " : Outport  SampleTime=1e-08
  wires:
  "a, b, c"/1 -> Reshape/1
  t1/1 -> delayMatch1/1
  select_2/1 -> delayMatch/1
  Gain2/1(Out1) -> "alpha, beta, 0 "/1
  delayMatch1/1 -> Gain2/2(In2)
  MMul_add_12/1(Out1) -> reshape_mmulResult/1
  MMul_add_01/1(Out1) -> MMul_add_12/1(In1)
  MMul_dot_product/1(Out1) -> reshape_dotProduct/1
  Gain2_const/1 -> t1/1, t1/2, t1/3
  Gain4_const/1 -> t/1
  delayMatch/1 -> MMul_add_12/2(In2)
  select_1/1 -> MMul_add_01/2(In2)
  select_0/1 -> MMul_add_01/1(In1)
  reshape_dotProduct/1 -> select_0/1, select_1/1, select_2/1
  Row2Col_in1/1 -> MMul_dot_product/2(In2)
  Row2Col_in0/1 -> MMul_dot_product/1(In1)
  select_indices1/1 -> Row2Col_in1/1
  select_indices0/1 -> Row2Col_in0/1
  vectorized_in0/1 -> select_indices0/1
  t/1 -> vectorized_in0/1
  Reshape/1 -> select_indices1/1
  reshape_mmulResult/1 -> Gain2/1(In1)

== system gm_uz_pmsm_model_9ph_vnl/uz_pmsm_model_9ph/Line-Line to Phase voltage1/alpha_beta_0   to   abc ==
  "alpha, beta, 0  " : Inport  OutDataTypeStr=single  PortDimensions=[3]  SampleTime=1e-08
  Gain4_const : Constant  Value=single([1 -0.5 -0.5 0 0.8660253882408142 -0.8660253882408142 1 1 1]).'  OutDataTypeStr=single  SampleTime=1e-08
  MMul_add_01 : Subsystem
      mask Display: disp('NFP\nadd');
  MMul_add_12 : Subsystem
      mask Display: disp('NFP\nadd');
  MMul_dot_product : Subsystem
      mask Display: disp('NFP\nmul');
  Reshape : Reshape  OutputDimensionality=Column vector (2-D)
  Row2Col_in0 : Reshape  OutputDimensionality=Column vector (2-D)
  Row2Col_in1 : Reshape  OutputDimensionality=Column vector (2-D)
  delayMatch : Delay  DelayLength=double(6)  InitialCondition=0  SampleTime=1e-08
  reshape_dotProduct : Reshape  OutputDimensionality=Customize  OutputDimensions=[3,3]
  reshape_mmulResult : Reshape  OutputDimensionality=Customize  OutputDimensions=[3,1]
  select_0 : Selector  NumberOfDimensions=2  SampleTime=1e-08  IndexOptions=Index vector (dialog),Select all  Indices=double(1),[]  OutputSizes=1
  select_1 : Selector  NumberOfDimensions=2  SampleTime=1e-08  IndexOptions=Index vector (dialog),Select all  Indices=double(2),[]  OutputSizes=1
  select_2 : Selector  NumberOfDimensions=2  SampleTime=1e-08  IndexOptions=Index vector (dialog),Select all  Indices=double(3),[]  OutputSizes=1
  select_indices0 : Selector  SampleTime=1e-08  IndexOptions=Index vector (dialog)  Indices=double([1 4 7 2 5 8 3 6 9])  OutputSizes=1
  select_indices1 : Selector  SampleTime=1e-08  IndexOptions=Index vector (dialog)  Indices=double([1 2 3 1 2 3 1 2 3])  OutputSizes=1
  t : Reshape  OutputDimensionality=Customize  OutputDimensions=[3,3]
  vectorized_in0 : Reshape  OutputDimensionality=Row vector (2-D)
  "a, b, c" : Outport  SampleTime=1e-08
  wires:
  "alpha, beta, 0  "/1 -> Reshape/1
  select_2/1 -> delayMatch/1
  MMul_add_12/1(Out1) -> reshape_mmulResult/1
  MMul_add_01/1(Out1) -> MMul_add_12/1(In1)
  MMul_dot_product/1(Out1) -> reshape_dotProduct/1
  Gain4_const/1 -> t/1
  delayMatch/1 -> MMul_add_12/2(In2)
  select_1/1 -> MMul_add_01/2(In2)
  select_0/1 -> MMul_add_01/1(In1)
  reshape_dotProduct/1 -> select_0/1, select_1/1, select_2/1
  Row2Col_in1/1 -> MMul_dot_product/2(In2)
  Row2Col_in0/1 -> MMul_dot_product/1(In1)
  select_indices1/1 -> Row2Col_in1/1
  select_indices0/1 -> Row2Col_in0/1
  vectorized_in0/1 -> select_indices0/1
  t/1 -> vectorized_in0/1
  Reshape/1 -> select_indices1/1
  reshape_mmulResult/1 -> "a, b, c"/1

== system gm_uz_pmsm_model_9ph_vnl/uz_pmsm_model_9ph/Line-Line to Phase voltage2/Product ==
  In1 : Inport
  In2 : Inport  Port=2
  Product : Product  Inputs=**  OutDataTypeStr=single  SampleTime=1e-08
  Product_pd1 : Delay  DelayLength=6
  Out1 : Outport
  wires:
  Product_pd1/1 -> Out1/1
  Product/1 -> Product_pd1/1
  In2/1 -> Product/2
  In1/1 -> Product/1

== system gm_uz_pmsm_model_9ph_vnl/uz_pmsm_model_9ph/Line-Line to Phase voltage2/Product1 ==
  In1 : Inport
  In2 : Inport  Port=2
  Product1 : Product  Inputs=**  OutDataTypeStr=single  SampleTime=1e-08
  Product1_pd1 : Delay  DelayLength=6
  Out1 : Outport
  wires:
  Product1_pd1/1 -> Out1/1
  Product1/1 -> Product1_pd1/1
  In2/1 -> Product1/2
  In1/1 -> Product1/1

== system gm_uz_pmsm_model_9ph_vnl/uz_pmsm_model_9ph/Line-Line to Phase voltage2/Product2 ==
  In1 : Inport
  In2 : Inport  Port=2
  Product2 : Product  Inputs=**  OutDataTypeStr=single  SampleTime=1e-08
  Product2_pd1 : Delay  DelayLength=6
  Out1 : Outport
  wires:
  Product2_pd1/1 -> Out1/1
  Product2/1 -> Product2_pd1/1
  In2/1 -> Product2/2
  In1/1 -> Product2/1

== system gm_uz_pmsm_model_9ph_vnl/uz_pmsm_model_9ph/Line-Line to Phase voltage2/Product3 ==
  In1 : Inport
  In2 : Inport  Port=2
  Product3 : Product  Inputs=**  OutDataTypeStr=single  SampleTime=1e-08
  Product3_pd1 : Delay  DelayLength=6
  Out1 : Outport
  wires:
  Product3_pd1/1 -> Out1/1
  Product3/1 -> Product3_pd1/1
  In2/1 -> Product3/2
  In1/1 -> Product3/1

== system gm_uz_pmsm_model_9ph_vnl/uz_pmsm_model_9ph/Line-Line to Phase voltage2/Product_AC_minus_BD ==
  In1 : Inport
  In2 : Inport  Port=2
  Product_AC_minus_BD : Sum  Inputs=+-  OutDataTypeStr=single  SampleTime=1e-08
  Product_AC_minus_BD_pd1 : Delay  DelayLength=6
  Out1 : Outport
  wires:
  Product_AC_minus_BD_pd1/1 -> Out1/1
  Product_AC_minus_BD/1 -> Product_AC_minus_BD_pd1/1
  In2/1 -> Product_AC_minus_BD/2
  In1/1 -> Product_AC_minus_BD/1

== system gm_uz_pmsm_model_9ph_vnl/uz_pmsm_model_9ph/Line-Line to Phase voltage2/Product_AD_plus_BC ==
  In1 : Inport
  In2 : Inport  Port=2
  Product_AD_plus_BC : Sum  OutDataTypeStr=single  SampleTime=1e-08
  Product_AD_plus_BC_pd1 : Delay  DelayLength=6
  Out1 : Outport
  wires:
  Product_AD_plus_BC_pd1/1 -> Out1/1
  Product_AD_plus_BC/1 -> Product_AD_plus_BC_pd1/1
  In2/1 -> Product_AD_plus_BC/2
  In1/1 -> Product_AD_plus_BC/1

== system gm_uz_pmsm_model_9ph_vnl/uz_pmsm_model_9ph/Line-Line to Phase voltage2/abc   to   alpha_beta_0 ==
  "a, b, c" : Inport  OutDataTypeStr=single  PortDimensions=[3]  SampleTime=1e-08
  Gain2 : Subsystem
      mask Display: disp('NFP\nmul');
  Gain2_const : Constant  Value=single(0.6666666865348816)  OutDataTypeStr=single  SampleTime=1e-08
  Gain4_const : Constant  Value=single([1 0 0.5 -0.5 0.8660253882408142 0.5 -0.5 -0.8660253882408142 0.5]).'  OutDataTypeStr=single  SampleTime=1e-08
  MMul_add_01 : Subsystem
      mask Display: disp('NFP\nadd');
  MMul_add_12 : Subsystem
      mask Display: disp('NFP\nadd');
  MMul_dot_product : Subsystem
      mask Display: disp('NFP\nmul');
  Reshape : Reshape  OutputDimensionality=Column vector (2-D)
  Row2Col_in0 : Reshape  OutputDimensionality=Column vector (2-D)
  Row2Col_in1 : Reshape  OutputDimensionality=Column vector (2-D)
  delayMatch : Delay  DelayLength=double(6)  InitialCondition=0  SampleTime=1e-08
  delayMatch1 : Delay  DelayLength=double(18)  InitialCondition=0  SampleTime=1e-08
  reshape_dotProduct : Reshape  OutputDimensionality=Customize  OutputDimensions=[3,3]
  reshape_mmulResult : Reshape  OutputDimensionality=Customize  OutputDimensions=[3,1]
  select_0 : Selector  NumberOfDimensions=2  SampleTime=1e-08  IndexOptions=Index vector (dialog),Select all  Indices=double(1),[]  OutputSizes=1
  select_1 : Selector  NumberOfDimensions=2  SampleTime=1e-08  IndexOptions=Index vector (dialog),Select all  Indices=double(2),[]  OutputSizes=1
  select_2 : Selector  NumberOfDimensions=2  SampleTime=1e-08  IndexOptions=Index vector (dialog),Select all  Indices=double(3),[]  OutputSizes=1
  select_indices0 : Selector  SampleTime=1e-08  IndexOptions=Index vector (dialog)  Indices=double([1 4 7 2 5 8 3 6 9])  OutputSizes=1
  select_indices1 : Selector  SampleTime=1e-08  IndexOptions=Index vector (dialog)  Indices=double([1 2 3 1 2 3 1 2 3])  OutputSizes=1
  t : Reshape  OutputDimensionality=Customize  OutputDimensions=[3,3]
  t1 : Mux  Inputs=3
  vectorized_in0 : Reshape  OutputDimensionality=Row vector (2-D)
  "alpha, beta, 0 " : Outport  SampleTime=1e-08
  wires:
  "a, b, c"/1 -> Reshape/1
  t1/1 -> delayMatch1/1
  select_2/1 -> delayMatch/1
  Gain2/1(Out1) -> "alpha, beta, 0 "/1
  delayMatch1/1 -> Gain2/2(In2)
  MMul_add_12/1(Out1) -> reshape_mmulResult/1
  MMul_add_01/1(Out1) -> MMul_add_12/1(In1)
  MMul_dot_product/1(Out1) -> reshape_dotProduct/1
  Gain2_const/1 -> t1/1, t1/2, t1/3
  Gain4_const/1 -> t/1
  delayMatch/1 -> MMul_add_12/2(In2)
  select_1/1 -> MMul_add_01/2(In2)
  select_0/1 -> MMul_add_01/1(In1)
  reshape_dotProduct/1 -> select_0/1, select_1/1, select_2/1
  Row2Col_in1/1 -> MMul_dot_product/2(In2)
  Row2Col_in0/1 -> MMul_dot_product/1(In1)
  select_indices1/1 -> Row2Col_in1/1
  select_indices0/1 -> Row2Col_in0/1
  vectorized_in0/1 -> select_indices0/1
  t/1 -> vectorized_in0/1
  Reshape/1 -> select_indices1/1
  reshape_mmulResult/1 -> Gain2/1(In1)

== system gm_uz_pmsm_model_9ph_vnl/uz_pmsm_model_9ph/Line-Line to Phase voltage2/alpha_beta_0   to   abc ==
  "alpha, beta, 0  " : Inport  OutDataTypeStr=single  PortDimensions=[3]  SampleTime=1e-08
  Gain4_const : Constant  Value=single([1 -0.5 -0.5 0 0.8660253882408142 -0.8660253882408142 1 1 1]).'  OutDataTypeStr=single  SampleTime=1e-08
  MMul_add_01 : Subsystem
      mask Display: disp('NFP\nadd');
  MMul_add_12 : Subsystem
      mask Display: disp('NFP\nadd');
  MMul_dot_product : Subsystem
      mask Display: disp('NFP\nmul');
  Reshape : Reshape  OutputDimensionality=Column vector (2-D)
  Row2Col_in0 : Reshape  OutputDimensionality=Column vector (2-D)
  Row2Col_in1 : Reshape  OutputDimensionality=Column vector (2-D)
  delayMatch : Delay  DelayLength=double(6)  InitialCondition=0  SampleTime=1e-08
  reshape_dotProduct : Reshape  OutputDimensionality=Customize  OutputDimensions=[3,3]
  reshape_mmulResult : Reshape  OutputDimensionality=Customize  OutputDimensions=[3,1]
  select_0 : Selector  NumberOfDimensions=2  SampleTime=1e-08  IndexOptions=Index vector (dialog),Select all  Indices=double(1),[]  OutputSizes=1
  select_1 : Selector  NumberOfDimensions=2  SampleTime=1e-08  IndexOptions=Index vector (dialog),Select all  Indices=double(2),[]  OutputSizes=1
  select_2 : Selector  NumberOfDimensions=2  SampleTime=1e-08  IndexOptions=Index vector (dialog),Select all  Indices=double(3),[]  OutputSizes=1
  select_indices0 : Selector  SampleTime=1e-08  IndexOptions=Index vector (dialog)  Indices=double([1 4 7 2 5 8 3 6 9])  OutputSizes=1
  select_indices1 : Selector  SampleTime=1e-08  IndexOptions=Index vector (dialog)  Indices=double([1 2 3 1 2 3 1 2 3])  OutputSizes=1
  t : Reshape  OutputDimensionality=Customize  OutputDimensions=[3,3]
  vectorized_in0 : Reshape  OutputDimensionality=Row vector (2-D)
  "a, b, c" : Outport  SampleTime=1e-08
  wires:
  "alpha, beta, 0  "/1 -> Reshape/1
  select_2/1 -> delayMatch/1
  MMul_add_12/1(Out1) -> reshape_mmulResult/1
  MMul_add_01/1(Out1) -> MMul_add_12/1(In1)
  MMul_dot_product/1(Out1) -> reshape_dotProduct/1
  Gain4_const/1 -> t/1
  delayMatch/1 -> MMul_add_12/2(In2)
  select_1/1 -> MMul_add_01/2(In2)
  select_0/1 -> MMul_add_01/1(In1)
  reshape_dotProduct/1 -> select_0/1, select_1/1, select_2/1
  Row2Col_in1/1 -> MMul_dot_product/2(In2)
  Row2Col_in0/1 -> MMul_dot_product/1(In1)
  select_indices1/1 -> Row2Col_in1/1
  select_indices0/1 -> Row2Col_in0/1
  vectorized_in0/1 -> select_indices0/1
  t/1 -> vectorized_in0/1
  Reshape/1 -> select_indices1/1
  reshape_mmulResult/1 -> "a, b, c"/1

== system gm_uz_pmsm_model_9ph_vnl/uz_pmsm_model_9ph/Transformation/Add ==
  In1 : Inport
  In2 : Inport  Port=2
  Add : Sum  OutDataTypeStr=single  SampleTime=1e-08
  Add_pd1 : Delay  DelayLength=6
  Out1 : Outport
  wires:
  Add_pd1/1 -> Out1/1
  Add/1 -> Add_pd1/1
  In2/1 -> Add/2
  In1/1 -> Add/1

== system gm_uz_pmsm_model_9ph_vnl/uz_pmsm_model_9ph/Transformation/Add1 ==
  In1 : Inport
  In2 : Inport  Port=2
  Add1 : Sum  Inputs=+-  OutDataTypeStr=single  SampleTime=1e-08
  Add1_pd1 : Delay  DelayLength=6
  Out1 : Outport
  wires:
  Add1_pd1/1 -> Out1/1
  Add1/1 -> Add1_pd1/1
  In2/1 -> Add1/2
  In1/1 -> Add1/1

== system gm_uz_pmsm_model_9ph_vnl/uz_pmsm_model_9ph/Transformation/Data Type Conversion39 ==
  In1 : Inport
  Data Type Conversion39 : DataTypeConversion  OutDataTypeStr=single  RndMeth=Nearest  SampleTime=1e-08
  Data Type Conversion39_pd1 : Delay  DelayLength=6
  Out1 : Outport
  wires:
  Data Type Conversion39_pd1/1 -> Out1/1
  Data Type Conversion39/1 -> Data Type Conversion39_pd1/1
  In1/1 -> Data Type Conversion39/1

== system gm_uz_pmsm_model_9ph_vnl/uz_pmsm_model_9ph/Transformation/Divide ==
  In1 : Inport
  In2 : Inport  Port=2
  Divide : Product  Inputs=**  OutDataTypeStr=single  SampleTime=1e-08
  Divide_pd1 : Delay  DelayLength=6
  Out1 : Outport
  wires:
  Divide_pd1/1 -> Out1/1
  Divide/1 -> Divide_pd1/1
  In2/1 -> Divide/2
  In1/1 -> Divide/1

== system gm_uz_pmsm_model_9ph_vnl/uz_pmsm_model_9ph/Transformation/Divide1 ==
  In1 : Inport
  In2 : Inport  Port=2
  Divide1 : Product  Inputs=**  OutDataTypeStr=single  SampleTime=1e-08
  Divide1_pd1 : Delay  DelayLength=6
  Out1 : Outport
  wires:
  Divide1_pd1/1 -> Out1/1
  Divide1/1 -> Divide1_pd1/1
  In2/1 -> Divide1/2
  In1/1 -> Divide1/1

== system gm_uz_pmsm_model_9ph_vnl/uz_pmsm_model_9ph/Transformation/Divide2 ==
  In1 : Inport
  In2 : Inport  Port=2
  Divide2 : Product  Inputs=**  OutDataTypeStr=single  SampleTime=1e-08
  Divide2_pd1 : Delay  DelayLength=6
  Out1 : Outport
  wires:
  Divide2_pd1/1 -> Out1/1
  Divide2/1 -> Divide2_pd1/1
  In2/1 -> Divide2/2
  In1/1 -> Divide2/1

== system gm_uz_pmsm_model_9ph_vnl/uz_pmsm_model_9ph/Transformation/Divide3 ==
  In1 : Inport
  In2 : Inport  Port=2
  Divide3 : Product  Inputs=**  OutDataTypeStr=single  SampleTime=1e-08
  Divide3_pd1 : Delay  DelayLength=6
  Out1 : Outport
  wires:
  Divide3_pd1/1 -> Out1/1
  Divide3/1 -> Divide3_pd1/1
  In2/1 -> Divide3/2
  In1/1 -> Divide3/1

== system gm_uz_pmsm_model_9ph_vnl/uz_pmsm_model_9ph/Transformation/t3 ==
  in0 : Inport
  ColVec1 : Selector  NumberOfDimensions=2  IndexOptions=Select all,Index vector (dialog)  Indices=1,1  OutputSizes=1,1
  ColVec2 : Selector  NumberOfDimensions=2  IndexOptions=Select all,Index vector (dialog)  Indices=1,2  OutputSizes=1,1
  ColVec3 : Selector  NumberOfDimensions=2  IndexOptions=Select all,Index vector (dialog)  Indices=1,3  OutputSizes=1,1
  ColVec4 : Selector  NumberOfDimensions=2  IndexOptions=Select all,Index vector (dialog)  Indices=1,4  OutputSizes=1,1
  ColVec5 : Selector  NumberOfDimensions=2  IndexOptions=Select all,Index vector (dialog)  Indices=1,5  OutputSizes=1,1
  ColVec6 : Selector  NumberOfDimensions=2  IndexOptions=Select all,Index vector (dialog)  Indices=1,6  OutputSizes=1,1
  ColVec7 : Selector  NumberOfDimensions=2  IndexOptions=Select all,Index vector (dialog)  Indices=1,7  OutputSizes=1,1
  ColVec8 : Selector  NumberOfDimensions=2  IndexOptions=Select all,Index vector (dialog)  Indices=1,8  OutputSizes=1,1
  ColVec9 : Selector  NumberOfDimensions=2  IndexOptions=Select all,Index vector (dialog)  Indices=1,9  OutputSizes=1,1
  out0 : Outport
  out1 : Outport  Port=2
  out2 : Outport  Port=3
  out3 : Outport  Port=4
  out4 : Outport  Port=5
  out5 : Outport  Port=6
  out6 : Outport  Port=7
  out7 : Outport  Port=8
  out8 : Outport  Port=9
  wires:
  ColVec9/1 -> out8/1
  ColVec8/1 -> out7/1
  ColVec7/1 -> out6/1
  ColVec6/1 -> out5/1
  ColVec5/1 -> out4/1
  ColVec4/1 -> out3/1
  ColVec3/1 -> out2/1
  ColVec2/1 -> out1/1
  ColVec1/1 -> out0/1
  in0/1 -> ColVec9/1, ColVec8/1, ColVec7/1, ColVec6/1, ColVec5/1, ColVec4/1, ColVec3/1, ColVec2/1, ColVec1/1

== system gm_uz_pmsm_model_9ph_vnl/uz_pmsm_model_9ph/Transformation1/Add ==
  In1 : Inport
  In2 : Inport  Port=2
  Add : Sum  Inputs=+-  OutDataTypeStr=single  SampleTime=1e-08
  Add_pd1 : Delay  DelayLength=6
  Out1 : Outport
  wires:
  Add_pd1/1 -> Out1/1
  Add/1 -> Add_pd1/1
  In2/1 -> Add/2
  In1/1 -> Add/1

== system gm_uz_pmsm_model_9ph_vnl/uz_pmsm_model_9ph/Transformation1/Add1 ==
  In1 : Inport
  In2 : Inport  Port=2
  Add1 : Sum  OutDataTypeStr=single  SampleTime=1e-08
  Add1_pd1 : Delay  DelayLength=6
  Out1 : Outport
  wires:
  Add1_pd1/1 -> Out1/1
  Add1/1 -> Add1_pd1/1
  In2/1 -> Add1/2
  In1/1 -> Add1/1

== system gm_uz_pmsm_model_9ph_vnl/uz_pmsm_model_9ph/Transformation1/Data Type Conversion28 ==
  In1 : Inport
  Data Type Conversion28 : DataTypeConversion  OutDataTypeStr=fixdt(1, 25, 12)  RndMeth=Nearest  SampleTime=1e-08
  Data Type Conversion28_pd1 : Delay  DelayLength=6
  Out1 : Outport
  wires:
  Data Type Conversion28_pd1/1 -> Out1/1
  Data Type Conversion28/1 -> Data Type Conversion28_pd1/1
  In1/1 -> Data Type Conversion28/1
